simulink model "NewTapWithdrawalCircuit"  (R2016b)
settings: Solver=VariableStepAuto  StartTime=0.0  StopTime=30  RelTol=1e-3  EnableMultiTasking=on
(part 1 of 2)
settings Model: Creator=ramin  LastModifiedBy=ramin
settings DataIOCC: LimitDataPoints=on
settings OptimizationCC: LifeSpan=inf
settings DebuggingCC: AllowSymbolicDim=off  SFUnexpectedBacktrackingDiag=warning  SFNoUnconditionalDefaultTransitionDiag=warning  SFExecutionAtInitializationDiag=none
settings ModelReferenceCC: PropagateSignalLabelsOutOfModel=off
settings GRTTargetCC: TargetLangStandard=C89/C90 (ANSI)
settings ConfigComp: CovMetricSettings=dw  CovHtmlReporting=on  CovSaveCumulativeToWorkspaceVar=on  CovSaveSingleToWorkspaceVar=on  CovExternalEMLEnable=off

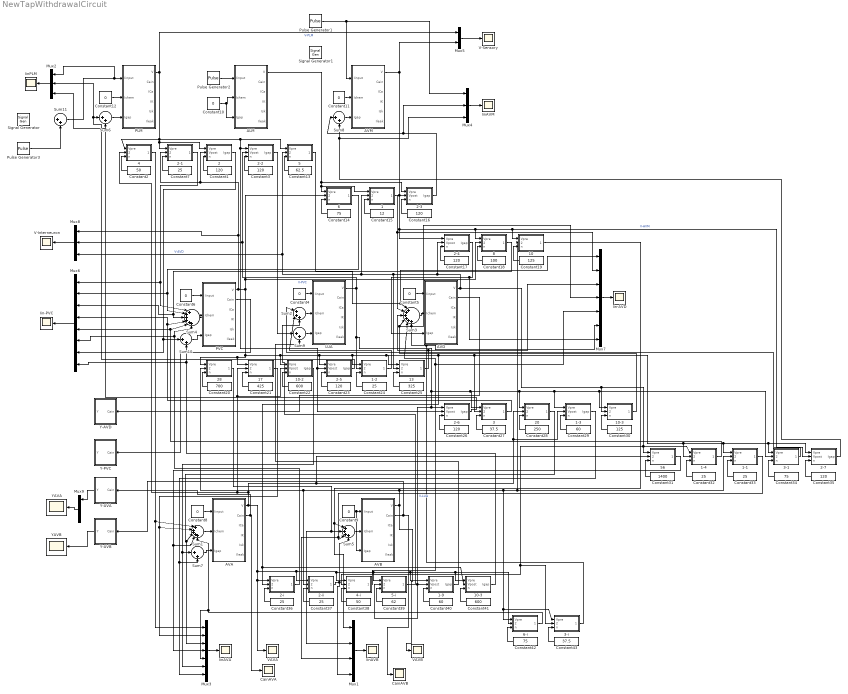
== system NewTapWithdrawalCircuit ==
  1 : Subsystem
  1-1 : Subsystem
  1-2 : Subsystem
  "1-3 " : Subsystem
  1-4 : Subsystem
  1-9 : Subsystem
  10 : Subsystem
  10-2 : Subsystem
  10-3 : Subsystem
  "10-3 " : Subsystem
  13 : Subsystem
  17 : Subsystem
  2 : Subsystem
  2-1 : Subsystem
  2-2 : Subsystem
  2-3 : Subsystem
  2-4 : Subsystem
  2-5 : Subsystem
  2-6 : Subsystem
  2-7 : Subsystem
  2-i : Subsystem
  2-ii : Subsystem
  20 : Subsystem
  28 : Subsystem
  3 : Subsystem
  3-1 : Subsystem
  3-i : Subsystem
  4 : Subsystem
  4-i : Subsystem
  5 : Subsystem
  5-i : Subsystem
  56 : Subsystem
  6 : Subsystem
  6-i : Subsystem
  8 : Subsystem
  ALM : Subsystem
  AVA : Subsystem
  AVB : Subsystem
  AVD : Subsystem
  AVM : Subsystem
  CainAVA : Scope
  CainAVB : Scope
  Constant{1,3,16..17,23,26,35} (7 alike) : Constant  Value=120
  Constant{4..6,8..12} (8 alike) : Constant  Value=0
  Constant13 : Constant  Value=62.5
  Constant14 : Constant  Value=75
  Constant15 : Constant  Value=12
  Constant18 : Constant  Value=100
  Constant19 : Constant  Value=125
  Constant2 : Constant  Value=50
  Constant20 : Constant  Value=700
  Constant21 : Constant  Value=425
  Constant22 : Constant  Value=600
  Constant{7,24,32..33,36..37} (6 alike) : Constant  Value=25
  Constant25 : Constant  Value=325
  Constant27 : Constant  Value=37.5
  Constant28 : Constant  Value=250
  Constant29 : Constant  Value=60
  Constant30 : Constant  Value=125
  Constant31 : Constant  Value=1400
  Constant34 : Constant  Value=75
  Constant38 : Constant  Value=50
  Constant39 : Constant  Value=62
  Constant40 : Constant  Value=60
  Constant41 : Constant  Value=600
  Constant42 : Constant  Value=75
  Constant43 : Constant  Value=37.5
  Iin-AVD : Scope
  Iin-PVC : Scope
  IinAVA : Scope
  IinAVB : Scope
  IinAVM : Scope
  IinPLM : Scope
  LUA : Subsystem
  Mux1 : Mux
  Mux2 : Mux  Inputs=3
  Mux3 : Mux  Inputs=7
  Mux4 : Mux  Inputs=3
  Mux5 : Mux  Inputs=2
  Mux6 : Mux  Inputs=8
  Mux7 : Mux  Inputs=7
  Mux8 : Mux  Inputs=3
  Mux9 : Mux
  PLM : Subsystem
  PVC : Subsystem
  Pulse Generator1 : DiscretePulseGenerator  PulseType=Time based  Amplitude=10000  Period=20  PulseWidth=30  PhaseDelay=2
  Pulse Generator2 : DiscretePulseGenerator  PulseType=Time based  Amplitude=0  Period=12  PulseWidth=30  PhaseDelay=2
  Pulse Generator3 : DiscretePulseGenerator  PulseType=Time based  Amplitude=0  Period=12  PulseWidth=30  PhaseDelay=2
  Signal Generator : SignalGenerator  WaveForm=random  Amplitude=50000  Frequency=500
  Signal Generator1 : SignalGenerator  WaveForm=random  Amplitude=50000  Frequency=500
  Sum1 : Sum  Inputs=|+++++
  Sum{6..11} (6 alike) : Sum  Inputs=|++
  Sum2 : Sum  Inputs=|+++
  Sum3 : Sum  Inputs=|++++++
  Sum4 : Sum  Inputs=|++++++
  Sum5 : Sum  Inputs=|++++
  V-Interneuron : Scope
  V-Sensory : Scope
  VAVA : Scope
  VAVB : Scope
  Y-AVA : Subsystem
  Y-AVB : Subsystem
  Y-AVD : Subsystem
  Y-PVC : Subsystem
  YAVA : Scope
  YAVB : Scope
  wires:
  Constant7/1 -> 2-1/3(n)
  Sum4/1 -> PVC/2(Ichem)
  2-1/1(Ichem) -> Sum4/1, Mux6/1
  Constant1/1 -> 2/3(n)
  2/1(Igap) -> Mux6/7, Sum10/1
  Constant2/1 -> 4/3(n)
  Sum1/1 -> AVA/2(Ichem)
  4/1(Ichem) -> Mux3/1, Sum1/1
  LUA/1(V) -> Mux8/2, 2-2/2(Vpost), 5-i/2(Vpost), 1-9/2(Vpost), 2-6/1(Vpre), 20/1(Vpre), 3-1/2(Vpost), "10-3 "/1(Vpre), "1-3 "/1(Vpre), 3/1(Vpre), 1-2/2(Vpost)  "V-LUA"
  Sum2/1 -> LUA/2(Ichem)
  2-2/1(Igap) -> Sum9/1
  Constant3/1 -> 2-2/3(n)
  Sum11/1 -> Mux2/1, PLM/1(Iinput)
  Sum3/1 -> AVD/2(Ichem)
  5/1(Ichem) -> Mux7/1, Sum3/1
  Constant5/1 -> AVD/1(Iinput)
  Constant4/1 -> LUA/1(Iinput)
  Constant6/1 -> PVC/1(Iinput)
  Constant8/1 -> AVA/1(Iinput)
  Constant9/1 -> AVB/3(Igap), AVB/1(Iinput)
  Pulse Generator2/1 -> ALM/1(Iinput)
  Constant11/1 -> AVM/2(Ichem)
  Constant12/1 -> PLM/2(Ichem)
  Sum5/1 -> AVB/2(Ichem)
  Constant13/1 -> 5/3(n)
  ALM/1(V) -> 2-3/1(Vpre), 1/1(Vpre), 6/1(Vpre)
  6/1(Ichem) -> Sum4/2, Mux6/2
  Constant14/1 -> 6/3(n)
  1/1(Ichem) -> Sum3/2, Mux7/2
  Constant15/1 -> 1/3(n)
  Constant16/1 -> 2-3/3(n)
  AVM/1(V) -> 2-7/2(Vpost), 10/1(Vpre), 8/1(Vpre), 2-4/1(Vpre), 2-3/2(Vpost), Mux5/2  "V-AVM"
  Constant17/1 -> 2-4/3(n)
  2-4/1(Igap) -> Mux7/7, AVD/3(Igap)
  Constant18/1 -> 8/3(n)
  8/1(Ichem) -> Sum4/3, Mux6/3
  Constant19/1 -> 10/3(n)
  10/1(Ichem) -> Mux1/1, Sum5/1
  AVB/1(V) -> 2-ii/2(Vpost), 28/2(Vpost), 3-i/1(Vpre), 6-i/1(Vpre), 1-1/2(Vpost), 10/2(Vpost), VAVB/1
  Constant20/1 -> 28/3(n)
  28/1(Ichem) -> Sum5/2, Mux1/2
  Constant21/1 -> 17/3(n)
  17/1(Ichem) -> Mux3/2, Sum1/2
  Constant22/1 -> 10-2/3(n)
  10-2/1(Igap) -> Mux3/6, Sum7/1
  PLM/1(V) -> 2-2/1(Vpre), 2-6/2(Vpost), 2-5/2(Vpost), 5/1(Vpre), 4/1(Vpre), 2-1/1(Vpre), 2/1(Vpre), Mux5/1  "V-PLM"
  Constant23/1 -> 2-5/3(n)
  2-5/1(Igap) -> Mux2/2, Sum6/1
  Constant24/1 -> 1-2/3(n)
  1-2/1(Ichem) -> Sum2/2
  Constant25/1 -> 13/3(n)
  Constant26/1 -> 2-6/3(n)
  2-6/1(Igap) -> Mux2/3, Sum6/2
  Constant27/1 -> 3/3(n)
  3/1(Ichem) -> Mux6/4, Sum4/4
  Constant28/1 -> 20/3(n)
  20/1(Ichem) -> Sum1/3, Mux3/3
  Constant29/1 -> "1-3 "/3(n)
  "1-3 "/1(Igap) -> Mux3/7, Sum7/2
  Sum7/1 -> AVA/3(Igap)
  Constant30/1 -> "10-3 "/3(n)
  "10-3 "/1(Ichem) -> Mux7/4, Sum3/4
  AVA/1(V) -> 56/2(Vpost), "1-3 "/2(Vpost), 20/2(Vpost), 10-2/2(Vpost), 17/2(Vpost), 4/2(Vpost), 2-ii/1(Vpre), 4-i/1(Vpre), 5-i/1(Vpre), 1-9/1(Vpre), 6-i/2(Vpost), 10-3/1(Vpre), 2-i/1(Vpre), VAVA/1
  Constant31/1 -> 56/3(n)
  56/1(Ichem) -> Mux3/4, Sum1/4
  1-4/1(Ichem) -> Mux6/5, Sum4/5
  Constant32/1 -> 1-4/3(n)
  Constant33/1 -> 1-1/3(n)
  1-1/1(Ichem) -> Mux1/3, Sum5/3
  Constant34/1 -> 3-1/3(n)
  3-1/1(Ichem) -> Sum2/1
  Sum6/1 -> PLM/3(Igap)
  Sum8/1 -> AVM/3(Igap)
  Constant35/1 -> 2-7/3(n)
  2-7/1(Igap) -> Mux4/3, Sum8/2
  Constant36/1 -> 2-i/3(n)
  2-i/1(Ichem) -> Mux6/6, Sum4/6
  Constant37/1 -> 2-ii/3(n)
  2-ii/1(Ichem) -> Mux1/4, Sum5/4
  Constant38/1 -> 4-i/3(n)
  4-i/1(Ichem) -> Mux7/5, Sum3/5
  5-i/1(Ichem) -> Sum2/3
  Constant39/1 -> 5-i/3(n)
  Sum9/1 -> LUA/3(Igap)
  1-9/1(Igap) -> Sum9/2
  Constant40/1 -> 1-9/3(n)
  Constant41/1 -> 10-3/3(n)
  Sum10/1 -> PVC/3(Igap)
  10-3/1(Igap) -> Sum10/2, Mux6/8
  Constant42/1 -> 6-i/3(n)
  6-i/1(Ichem) -> Mux3/5, Sum1/5
  3-i/1(Ichem) -> Sum3/6, Mux7/6
  Constant43/1 -> 3-i/3(n)
  Mux3/1 -> IinAVA/1
  Mux1/1 -> IinAVB/1
  AVA/2("Cain ") -> Y-AVA/1(Cain), CainAVA/1
  AVB/2("Cain ") -> Y-AVB/1(Cain), CainAVB/1
  Constant10/1 -> ALM/3(Igap), ALM/2(Ichem)
  Mux2/1 -> IinPLM/1
  Mux4/1 -> IinAVM/1
  2-3/1(Igap) -> Mux4/2, Sum8/1
  Mux5/1 -> V-Sensory/1
  Mux6/1 -> Iin-PVC/1
  Mux7/1 -> Iin-AVD/1
  13/1(Ichem) -> Mux7/3, Sum3/3
  Mux8/1 -> V-Interneuron/1
  PVC/1(V) -> Mux8/1, 2-1/2(Vpost), 2/2(Vpost), 8/2(Vpost), 6/2(Vpost), 17/1(Vpre), 28/1(Vpre), 2-5/1(Vpre), 2-i/2(Vpost), 10-3/2(Vpost), 3/2(Vpost), 2-7/1(Vpre), 3-1/1(Vpre), 1-1/1(Vpre), 1-4/2(Vpost), 13/1(Vpre), 1-2/1(Vpre), 10-2/1(Vpre)  "V-PVC"
  AVD/1(V) -> 1-4/1(Vpre), 3-i/2(Vpost), 4-i/2(Vpost), 56/1(Vpre), "10-3 "/2(Vpost), 2-4/2(Vpost), 1/2(Vpost), Mux8/3, 5/2(Vpost), 13/2(Vpost)  "V-AVD"
  Y-AVA/1(Y) -> Mux9/1
  Y-AVB/1(Y) -> YAVB/1
  Mux9/1 -> YAVA/1
  PVC/2("Cain ") -> Y-PVC/1(Cain)
  AVD/2("Cain ") -> Y-AVD/1(Cain)
  Pulse Generator1/1 -> AVM/1(Iinput), Mux4/1
  Pulse Generator3/1 -> Sum11/2

== system NewTapWithdrawalCircuit/1 ==
  Vpre : Inport
  Vpost : Inport  Port=2
  n : Inport  Port=3
  Divide1 : Product  Inputs=*/
  Divide2 : Product  Inputs=*/
  Echem : Constant  Value=-90
  Product2 : Product
  Sum6 : Sum  Inputs=|+-
  Sum7 : Sum  Inputs=|++
  Sum8 : Sum  Inputs=|+-
  Vrange : Constant  Value=3
  Vshift : Constant  Value=-30
  betaK1 : Math  SaturateOnIntegerOverflow=on
  c111 : Constant
  Ichem : Outport
  wires:
  Echem/1 -> Sum6/1
  n/1 -> Product2/2
  Sum6/1 -> Product2/1
  Product2/1 -> Divide1/1
  betaK1/1 -> Sum7/1
  c111/1 -> Sum7/2
  Vshift/1 -> Sum8/1
  Vpre/1 -> Sum8/2  "vpre"
  Sum8/1 -> Divide2/1
  Vrange/1 -> Divide2/2
  Divide2/1 -> betaK1/1
  Sum7/1 -> Divide1/2
  Divide1/1 -> Ichem/1  "Ichem"
  Vpost/1 -> Sum6/2

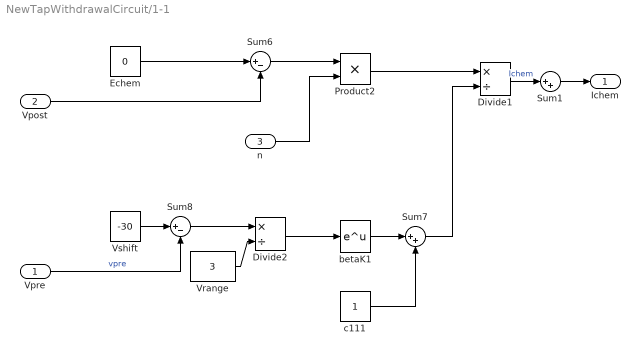
== system NewTapWithdrawalCircuit/1-1 ==
  Vpre : Inport
  Vpost : Inport  Port=2
  n : Inport  Port=3
  Divide1 : Product  Inputs=*/
  Divide2 : Product  Inputs=*/
  Echem : Constant  Value=0
  Product2 : Product
  Sum1 : Sum  Inputs=|++
  Sum6 : Sum  Inputs=|+-
  Sum7 : Sum  Inputs=|++
  Sum8 : Sum  Inputs=|+-
  Vrange : Constant  Value=3
  Vshift : Constant  Value=-30
  betaK1 : Math  SaturateOnIntegerOverflow=on
  c111 : Constant
  Ichem : Outport
  wires:
  Echem/1 -> Sum6/1
  n/1 -> Product2/2
  Sum6/1 -> Product2/1
  Product2/1 -> Divide1/1
  betaK1/1 -> Sum7/1
  c111/1 -> Sum7/2
  Vshift/1 -> Sum8/1
  Vpre/1 -> Sum8/2  "vpre"
  Sum8/1 -> Divide2/1
  Vrange/1 -> Divide2/2
  Divide2/1 -> betaK1/1
  Sum7/1 -> Divide1/2
  Divide1/1 -> Sum1/1  "Ichem"
  Vpost/1 -> Sum6/2
  Sum1/1 -> Ichem/1

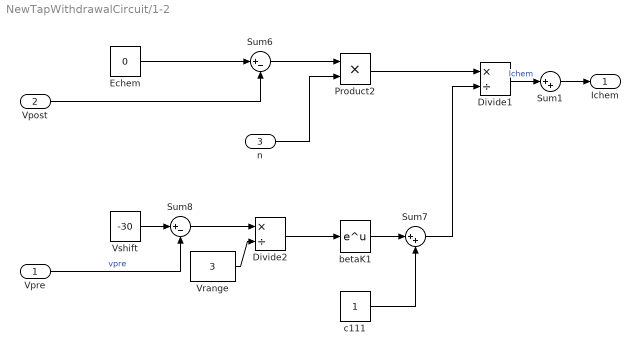
== system NewTapWithdrawalCircuit/1-2 ==
  Vpre : Inport
  Vpost : Inport  Port=2
  n : Inport  Port=3
  Divide1 : Product  Inputs=*/
  Divide2 : Product  Inputs=*/
  Echem : Constant  Value=0
  Product2 : Product
  Sum1 : Sum  Inputs=|++
  Sum6 : Sum  Inputs=|+-
  Sum7 : Sum  Inputs=|++
  Sum8 : Sum  Inputs=|+-
  Vrange : Constant  Value=3
  Vshift : Constant  Value=-30
  betaK1 : Math  SaturateOnIntegerOverflow=on
  c111 : Constant
  Ichem : Outport
  wires:
  Echem/1 -> Sum6/1
  n/1 -> Product2/2
  Sum6/1 -> Product2/1
  Product2/1 -> Divide1/1
  betaK1/1 -> Sum7/1
  c111/1 -> Sum7/2
  Vshift/1 -> Sum8/1
  Vpre/1 -> Sum8/2  "vpre"
  Sum8/1 -> Divide2/1
  Vrange/1 -> Divide2/2
  Divide2/1 -> betaK1/1
  Sum7/1 -> Divide1/2
  Divide1/1 -> Sum1/1  "Ichem"
  Vpost/1 -> Sum6/2
  Sum1/1 -> Ichem/1

== system NewTapWithdrawalCircuit/1-3  ==
  Vpre : Inport
  Vpost : Inport  Port=2
  n : Inport  Port=3
  Ggap : Constant  Value=1.02
  Product2 : Product  Inputs=3
  Sum6 : Sum  Inputs=|+-
  Igap : Outport
  wires:
  Vpre/1 -> Sum6/1
  n/1 -> Product2/2
  Sum6/1 -> Product2/1
  Product2/1 -> Igap/1  "Igap"
  Vpost/1 -> Sum6/2
  Ggap/1 -> Product2/3

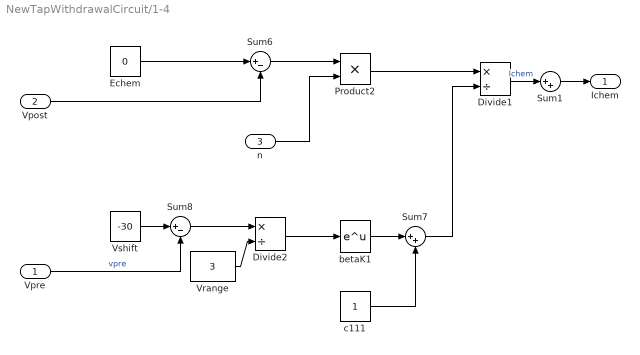
== system NewTapWithdrawalCircuit/1-4 ==
  Vpre : Inport
  Vpost : Inport  Port=2
  n : Inport  Port=3
  Divide1 : Product  Inputs=*/
  Divide2 : Product  Inputs=*/
  Echem : Constant  Value=0
  Product2 : Product
  Sum1 : Sum  Inputs=|++
  Sum6 : Sum  Inputs=|+-
  Sum7 : Sum  Inputs=|++
  Sum8 : Sum  Inputs=|+-
  Vrange : Constant  Value=3
  Vshift : Constant  Value=-30
  betaK1 : Math  SaturateOnIntegerOverflow=on
  c111 : Constant
  Ichem : Outport
  wires:
  Echem/1 -> Sum6/1
  n/1 -> Product2/2
  Sum6/1 -> Product2/1
  Product2/1 -> Divide1/1
  betaK1/1 -> Sum7/1
  c111/1 -> Sum7/2
  Vshift/1 -> Sum8/1
  Vpre/1 -> Sum8/2  "vpre"
  Sum8/1 -> Divide2/1
  Vrange/1 -> Divide2/2
  Divide2/1 -> betaK1/1
  Sum7/1 -> Divide1/2
  Divide1/1 -> Sum1/1  "Ichem"
  Vpost/1 -> Sum6/2
  Sum1/1 -> Ichem/1

== system NewTapWithdrawalCircuit/1-9 ==
  Vpre : Inport
  Vpost : Inport  Port=2
  n : Inport  Port=3
  Ggap : Constant  Value=1.02
  Product2 : Product  Inputs=3
  Sum6 : Sum  Inputs=|+-
  Igap : Outport
  wires:
  Vpre/1 -> Sum6/1
  n/1 -> Product2/2
  Sum6/1 -> Product2/1
  Product2/1 -> Igap/1  "Igap"
  Vpost/1 -> Sum6/2
  Ggap/1 -> Product2/3

== system NewTapWithdrawalCircuit/10 ==
  Vpre : Inport
  Vpost : Inport  Port=2
  n : Inport  Port=3
  Divide1 : Product  Inputs=*/
  Divide2 : Product  Inputs=*/
  Echem : Constant  Value=-90
  Product2 : Product
  Sum6 : Sum  Inputs=|+-
  Sum7 : Sum  Inputs=|++
  Sum8 : Sum  Inputs=|+-
  Vrange : Constant  Value=3
  Vshift : Constant  Value=-30
  betaK1 : Math  SaturateOnIntegerOverflow=on
  c111 : Constant
  Ichem : Outport
  wires:
  Echem/1 -> Sum6/1
  n/1 -> Product2/2
  Sum6/1 -> Product2/1
  Product2/1 -> Divide1/1
  betaK1/1 -> Sum7/1
  c111/1 -> Sum7/2
  Vshift/1 -> Sum8/1
  Vpre/1 -> Sum8/2  "vpre"
  Sum8/1 -> Divide2/1
  Vrange/1 -> Divide2/2
  Divide2/1 -> betaK1/1
  Sum7/1 -> Divide1/2
  Divide1/1 -> Ichem/1  "Ichem"
  Vpost/1 -> Sum6/2

== system NewTapWithdrawalCircuit/10-2 ==
  Vpre : Inport
  Vpost : Inport  Port=2
  n : Inport  Port=3
  Ggap : Constant  Value=1.02
  Product2 : Product  Inputs=3
  Sum6 : Sum  Inputs=|+-
  Igap : Outport
  wires:
  Vpre/1 -> Sum6/1
  n/1 -> Product2/2
  Sum6/1 -> Product2/1
  Product2/1 -> Igap/1  "Igap"
  Vpost/1 -> Sum6/2
  Ggap/1 -> Product2/3

== system NewTapWithdrawalCircuit/10-3 ==
  Vpre : Inport
  Vpost : Inport  Port=2
  n : Inport  Port=3
  Ggap : Constant  Value=1.02
  Product2 : Product  Inputs=3
  Sum6 : Sum  Inputs=|+-
  Igap : Outport
  wires:
  Vpre/1 -> Sum6/1
  n/1 -> Product2/2
  Sum6/1 -> Product2/1
  Product2/1 -> Igap/1  "Igap"
  Vpost/1 -> Sum6/2
  Ggap/1 -> Product2/3

== system NewTapWithdrawalCircuit/10-3  ==
  Vpre : Inport
  Vpost : Inport  Port=2
  n : Inport  Port=3
  Divide1 : Product  Inputs=*/
  Divide2 : Product  Inputs=*/
  Echem : Constant  Value=-90
  Product2 : Product
  Sum6 : Sum  Inputs=|+-
  Sum7 : Sum  Inputs=|++
  Sum8 : Sum  Inputs=|+-
  Vrange : Constant  Value=3
  Vshift : Constant  Value=-30
  betaK1 : Math  SaturateOnIntegerOverflow=on
  c111 : Constant
  Ichem : Outport
  wires:
  Echem/1 -> Sum6/1
  n/1 -> Product2/2
  Sum6/1 -> Product2/1
  Product2/1 -> Divide1/1
  betaK1/1 -> Sum7/1
  c111/1 -> Sum7/2
  Vshift/1 -> Sum8/1
  Vpre/1 -> Sum8/2  "vpre"
  Sum8/1 -> Divide2/1
  Vrange/1 -> Divide2/2
  Divide2/1 -> betaK1/1
  Sum7/1 -> Divide1/2
  Divide1/1 -> Ichem/1  "Ichem"
  Vpost/1 -> Sum6/2

== system NewTapWithdrawalCircuit/13 ==
  Vpre : Inport
  Vpost : Inport  Port=2
  n : Inport  Port=3
  Divide1 : Product  Inputs=*/
  Divide2 : Product  Inputs=*/
  Echem : Constant  Value=0
  Product2 : Product
  Sum1 : Sum  Inputs=|++
  Sum6 : Sum  Inputs=|+-
  Sum7 : Sum  Inputs=|++
  Sum8 : Sum  Inputs=|+-
  Vrange : Constant  Value=3
  Vshift : Constant  Value=-30
  betaK1 : Math  SaturateOnIntegerOverflow=on
  c111 : Constant
  Ichem : Outport
  wires:
  Echem/1 -> Sum6/1
  n/1 -> Product2/2
  Sum6/1 -> Product2/1
  Product2/1 -> Divide1/1
  betaK1/1 -> Sum7/1
  c111/1 -> Sum7/2
  Vshift/1 -> Sum8/1
  Vpre/1 -> Sum8/2  "vpre"
  Sum8/1 -> Divide2/1
  Vrange/1 -> Divide2/2
  Divide2/1 -> betaK1/1
  Sum7/1 -> Divide1/2
  Divide1/1 -> Sum1/1  "Ichem"
  Vpost/1 -> Sum6/2
  Sum1/1 -> Ichem/1

== system NewTapWithdrawalCircuit/17 ==
  Vpre : Inport
  Vpost : Inport  Port=2
  n : Inport  Port=3
  Divide1 : Product  Inputs=*/
  Divide2 : Product  Inputs=*/
  Echem : Constant  Value=0
  Product2 : Product
  Sum1 : Sum  Inputs=|++
  Sum6 : Sum  Inputs=|+-
  Sum7 : Sum  Inputs=|++
  Sum8 : Sum  Inputs=|+-
  Vrange : Constant  Value=3
  Vshift : Constant  Value=-30
  betaK1 : Math  SaturateOnIntegerOverflow=on
  c111 : Constant
  Ichem : Outport
  wires:
  Echem/1 -> Sum6/1
  n/1 -> Product2/2
  Sum6/1 -> Product2/1
  Product2/1 -> Divide1/1
  betaK1/1 -> Sum7/1
  c111/1 -> Sum7/2
  Vshift/1 -> Sum8/1
  Vpre/1 -> Sum8/2  "vpre"
  Sum8/1 -> Divide2/1
  Vrange/1 -> Divide2/2
  Divide2/1 -> betaK1/1
  Sum7/1 -> Divide1/2
  Divide1/1 -> Sum1/1  "Ichem"
  Vpost/1 -> Sum6/2
  Sum1/1 -> Ichem/1

== system NewTapWithdrawalCircuit/2 ==
  Vpre : Inport
  Vpost : Inport  Port=2
  n : Inport  Port=3
  Ggap : Constant  Value=1.02
  Product2 : Product  Inputs=3
  Sum6 : Sum  Inputs=|+-
  Igap : Outport
  wires:
  Vpre/1 -> Sum6/1
  n/1 -> Product2/2
  Sum6/1 -> Product2/1
  Product2/1 -> Igap/1  "Igap"
  Vpost/1 -> Sum6/2
  Ggap/1 -> Product2/3

== system NewTapWithdrawalCircuit/2-1 ==
  Vpre : Inport
  Vpost : Inport  Port=2
  n : Inport  Port=3
  Divide1 : Product  Inputs=*/
  Divide2 : Product  Inputs=*/
  Echem : Constant  Value=-90
  Product2 : Product
  Sum6 : Sum  Inputs=|+-
  Sum7 : Sum  Inputs=|++
  Sum8 : Sum  Inputs=|+-
  Vrange : Constant  Value=3
  Vshift : Constant  Value=-30
  betaK1 : Math  SaturateOnIntegerOverflow=on
  c111 : Constant
  Ichem : Outport
  wires:
  Echem/1 -> Sum6/1
  n/1 -> Product2/2
  Sum6/1 -> Product2/1
  Product2/1 -> Divide1/1
  betaK1/1 -> Sum7/1
  c111/1 -> Sum7/2
  Vshift/1 -> Sum8/1
  Vpre/1 -> Sum8/2  "vpre"
  Sum8/1 -> Divide2/1
  Vrange/1 -> Divide2/2
  Divide2/1 -> betaK1/1
  Sum7/1 -> Divide1/2
  Divide1/1 -> Ichem/1  "Ichem"
  Vpost/1 -> Sum6/2

== system NewTapWithdrawalCircuit/2-2 ==
  Vpre : Inport
  Vpost : Inport  Port=2
  n : Inport  Port=3
  Ggap : Constant  Value=1.02
  Product2 : Product  Inputs=3
  Sum6 : Sum  Inputs=|+-
  Igap : Outport
  wires:
  Vpre/1 -> Sum6/1
  n/1 -> Product2/2
  Sum6/1 -> Product2/1
  Product2/1 -> Igap/1  "Igap"
  Vpost/1 -> Sum6/2
  Ggap/1 -> Product2/3

== system NewTapWithdrawalCircuit/2-3 ==
  Vpre : Inport
  Vpost : Inport  Port=2
  n : Inport  Port=3
  Ggap : Constant  Value=1.02
  Product2 : Product  Inputs=3
  Sum6 : Sum  Inputs=|+-
  Igap : Outport
  wires:
  Vpre/1 -> Sum6/1
  n/1 -> Product2/2
  Sum6/1 -> Product2/1
  Product2/1 -> Igap/1  "Igap"
  Vpost/1 -> Sum6/2
  Ggap/1 -> Product2/3

== system NewTapWithdrawalCircuit/2-4 ==
  Vpre : Inport
  Vpost : Inport  Port=2
  n : Inport  Port=3
  Ggap : Constant  Value=1.02
  Product2 : Product  Inputs=3
  Sum6 : Sum  Inputs=|+-
  Igap : Outport
  wires:
  Vpre/1 -> Sum6/1
  n/1 -> Product2/2
  Sum6/1 -> Product2/1
  Product2/1 -> Igap/1  "Igap"
  Vpost/1 -> Sum6/2
  Ggap/1 -> Product2/3

== system NewTapWithdrawalCircuit/2-5 ==
  Vpre : Inport
  Vpost : Inport  Port=2
  n : Inport  Port=3
  Ggap : Constant  Value=1.02
  Product2 : Product  Inputs=3
  Sum6 : Sum  Inputs=|+-
  Igap : Outport
  wires:
  Vpre/1 -> Sum6/1
  n/1 -> Product2/2
  Sum6/1 -> Product2/1
  Product2/1 -> Igap/1  "Igap"
  Vpost/1 -> Sum6/2
  Ggap/1 -> Product2/3

== system NewTapWithdrawalCircuit/2-6 ==
  Vpre : Inport
  Vpost : Inport  Port=2
  n : Inport  Port=3
  Ggap : Constant  Value=1.02
  Product2 : Product  Inputs=3
  Sum6 : Sum  Inputs=|+-
  Igap : Outport
  wires:
  Vpre/1 -> Sum6/1
  n/1 -> Product2/2
  Sum6/1 -> Product2/1
  Product2/1 -> Igap/1  "Igap"
  Vpost/1 -> Sum6/2
  Ggap/1 -> Product2/3

== system NewTapWithdrawalCircuit/2-7 ==
  Vpre : Inport
  Vpost : Inport  Port=2
  n : Inport  Port=3
  Ggap : Constant  Value=1.02
  Product2 : Product  Inputs=3
  Sum6 : Sum  Inputs=|+-
  Igap : Outport
  wires:
  Vpre/1 -> Sum6/1
  n/1 -> Product2/2
  Sum6/1 -> Product2/1
  Product2/1 -> Igap/1  "Igap"
  Vpost/1 -> Sum6/2
  Ggap/1 -> Product2/3

== system NewTapWithdrawalCircuit/2-i ==
  Vpre : Inport
  Vpost : Inport  Port=2
  n : Inport  Port=3
  Divide1 : Product  Inputs=*/
  Divide2 : Product  Inputs=*/
  Echem : Constant  Value=-90
  Product2 : Product
  Sum6 : Sum  Inputs=|+-
  Sum7 : Sum  Inputs=|++
  Sum8 : Sum  Inputs=|+-
  Vrange : Constant  Value=3
  Vshift : Constant  Value=-30
  betaK1 : Math  SaturateOnIntegerOverflow=on
  c111 : Constant
  Ichem : Outport
  wires:
  Echem/1 -> Sum6/1
  n/1 -> Product2/2
  Sum6/1 -> Product2/1
  Product2/1 -> Divide1/1
  betaK1/1 -> Sum7/1
  c111/1 -> Sum7/2
  Vshift/1 -> Sum8/1
  Vpre/1 -> Sum8/2  "vpre"
  Sum8/1 -> Divide2/1
  Vrange/1 -> Divide2/2
  Divide2/1 -> betaK1/1
  Sum7/1 -> Divide1/2
  Divide1/1 -> Ichem/1  "Ichem"
  Vpost/1 -> Sum6/2

== system NewTapWithdrawalCircuit/2-ii ==
  Vpre : Inport
  Vpost : Inport  Port=2
  n : Inport  Port=3
  Divide1 : Product  Inputs=*/
  Divide2 : Product  Inputs=*/
  Echem : Constant  Value=-90
  Product2 : Product
  Sum6 : Sum  Inputs=|+-
  Sum7 : Sum  Inputs=|++
  Sum8 : Sum  Inputs=|+-
  Vrange : Constant  Value=3
  Vshift : Constant  Value=-30
  betaK1 : Math  SaturateOnIntegerOverflow=on
  c111 : Constant
  Ichem : Outport
  wires:
  Echem/1 -> Sum6/1
  n/1 -> Product2/2
  Sum6/1 -> Product2/1
  Product2/1 -> Divide1/1
  betaK1/1 -> Sum7/1
  c111/1 -> Sum7/2
  Vshift/1 -> Sum8/1
  Vpre/1 -> Sum8/2  "vpre"
  Sum8/1 -> Divide2/1
  Vrange/1 -> Divide2/2
  Divide2/1 -> betaK1/1
  Sum7/1 -> Divide1/2
  Divide1/1 -> Ichem/1  "Ichem"
  Vpost/1 -> Sum6/2

== system NewTapWithdrawalCircuit/20 ==
  Vpre : Inport
  Vpost : Inport  Port=2
  n : Inport  Port=3
  Divide1 : Product  Inputs=*/
  Divide2 : Product  Inputs=*/
  Echem : Constant  Value=-90
  Product2 : Product
  Sum6 : Sum  Inputs=|+-
  Sum7 : Sum  Inputs=|++
  Sum8 : Sum  Inputs=|+-
  Vrange : Constant  Value=3
  Vshift : Constant  Value=-30
  betaK1 : Math  SaturateOnIntegerOverflow=on
  c111 : Constant
  Ichem : Outport
  wires:
  Echem/1 -> Sum6/1
  n/1 -> Product2/2
  Sum6/1 -> Product2/1
  Product2/1 -> Divide1/1
  betaK1/1 -> Sum7/1
  c111/1 -> Sum7/2
  Vshift/1 -> Sum8/1
  Vpre/1 -> Sum8/2  "vpre"
  Sum8/1 -> Divide2/1
  Vrange/1 -> Divide2/2
  Divide2/1 -> betaK1/1
  Sum7/1 -> Divide1/2
  Divide1/1 -> Ichem/1  "Ichem"
  Vpost/1 -> Sum6/2

== system NewTapWithdrawalCircuit/28 ==
  Vpre : Inport
  Vpost : Inport  Port=2
  n : Inport  Port=3
  Divide1 : Product  Inputs=*/
  Divide2 : Product  Inputs=*/
  Echem : Constant  Value=0
  Product2 : Product
  Sum1 : Sum  Inputs=|++
  Sum6 : Sum  Inputs=|+-
  Sum7 : Sum  Inputs=|++
  Sum8 : Sum  Inputs=|+-
  Vrange : Constant  Value=3
  Vshift : Constant  Value=-30
  betaK1 : Math  SaturateOnIntegerOverflow=on
  c111 : Constant
  Ichem : Outport
  wires:
  Echem/1 -> Sum6/1
  n/1 -> Product2/2
  Sum6/1 -> Product2/1
  Product2/1 -> Divide1/1
  betaK1/1 -> Sum7/1
  c111/1 -> Sum7/2
  Vshift/1 -> Sum8/1
  Vpre/1 -> Sum8/2  "vpre"
  Sum8/1 -> Divide2/1
  Vrange/1 -> Divide2/2
  Divide2/1 -> betaK1/1
  Sum7/1 -> Divide1/2
  Divide1/1 -> Sum1/1  "Ichem"
  Vpost/1 -> Sum6/2
  Sum1/1 -> Ichem/1

== system NewTapWithdrawalCircuit/3 ==
  Vpre : Inport
  Vpost : Inport  Port=2
  n : Inport  Port=3
  Divide1 : Product  Inputs=*/
  Divide2 : Product  Inputs=*/
  Echem : Constant  Value=-90
  Product2 : Product
  Sum6 : Sum  Inputs=|+-
  Sum7 : Sum  Inputs=|++
  Sum8 : Sum  Inputs=|+-
  Vrange : Constant  Value=3
  Vshift : Constant  Value=-30
  betaK1 : Math  SaturateOnIntegerOverflow=on
  c111 : Constant
  Ichem : Outport
  wires:
  Echem/1 -> Sum6/1
  n/1 -> Product2/2
  Sum6/1 -> Product2/1
  Product2/1 -> Divide1/1
  betaK1/1 -> Sum7/1
  c111/1 -> Sum7/2
  Vshift/1 -> Sum8/1
  Vpre/1 -> Sum8/2  "vpre"
  Sum8/1 -> Divide2/1
  Vrange/1 -> Divide2/2
  Divide2/1 -> betaK1/1
  Sum7/1 -> Divide1/2
  Divide1/1 -> Ichem/1  "Ichem"
  Vpost/1 -> Sum6/2

== system NewTapWithdrawalCircuit/3-1 ==
  Vpre : Inport
  Vpost : Inport  Port=2
  n : Inport  Port=3
  Divide1 : Product  Inputs=*/
  Divide2 : Product  Inputs=*/
  Echem : Constant  Value=0
  Product2 : Product
  Sum1 : Sum  Inputs=|++
  Sum6 : Sum  Inputs=|+-
  Sum7 : Sum  Inputs=|++
  Sum8 : Sum  Inputs=|+-
  Vrange : Constant  Value=3
  Vshift : Constant  Value=-30
  betaK1 : Math  SaturateOnIntegerOverflow=on
  c111 : Constant
  Ichem : Outport
  wires:
  Echem/1 -> Sum6/1
  n/1 -> Product2/2
  Sum6/1 -> Product2/1
  Product2/1 -> Divide1/1
  betaK1/1 -> Sum7/1
  c111/1 -> Sum7/2
  Vshift/1 -> Sum8/1
  Vpre/1 -> Sum8/2  "vpre"
  Sum8/1 -> Divide2/1
  Vrange/1 -> Divide2/2
  Divide2/1 -> betaK1/1
  Sum7/1 -> Divide1/2
  Divide1/1 -> Sum1/1  "Ichem"
  Vpost/1 -> Sum6/2
  Sum1/1 -> Ichem/1

== system NewTapWithdrawalCircuit/3-i ==
  Vpre : Inport
  Vpost : Inport  Port=2
  n : Inport  Port=3
  Divide1 : Product  Inputs=*/
  Divide2 : Product  Inputs=*/
  Echem : Constant  Value=-90
  Product2 : Product
  Sum6 : Sum  Inputs=|+-
  Sum7 : Sum  Inputs=|++
  Sum8 : Sum  Inputs=|+-
  Vrange : Constant  Value=3
  Vshift : Constant  Value=-30
  betaK1 : Math  SaturateOnIntegerOverflow=on
  c111 : Constant
  Ichem : Outport
  wires:
  Echem/1 -> Sum6/1
  n/1 -> Product2/2
  Sum6/1 -> Product2/1
  Product2/1 -> Divide1/1
  betaK1/1 -> Sum7/1
  c111/1 -> Sum7/2
  Vshift/1 -> Sum8/1
  Vpre/1 -> Sum8/2  "vpre"
  Sum8/1 -> Divide2/1
  Vrange/1 -> Divide2/2
  Divide2/1 -> betaK1/1
  Sum7/1 -> Divide1/2
  Divide1/1 -> Ichem/1  "Ichem"
  Vpost/1 -> Sum6/2

== system NewTapWithdrawalCircuit/4 ==
  Vpre : Inport
  Vpost : Inport  Port=2
  n : Inport  Port=3
  Divide1 : Product  Inputs=*/
  Divide2 : Product  Inputs=*/
  Echem : Constant  Value=-90
  Product2 : Product
  Sum6 : Sum  Inputs=|+-
  Sum7 : Sum  Inputs=|++
  Sum8 : Sum  Inputs=|+-
  Vrange : Constant  Value=3
  Vshift : Constant  Value=-30
  betaK1 : Math  SaturateOnIntegerOverflow=on
  c111 : Constant
  Ichem : Outport
  wires:
  Echem/1 -> Sum6/1
  n/1 -> Product2/2
  Sum6/1 -> Product2/1
  Product2/1 -> Divide1/1
  betaK1/1 -> Sum7/1
  c111/1 -> Sum7/2
  Vshift/1 -> Sum8/1
  Vpre/1 -> Sum8/2  "vpre"
  Sum8/1 -> Divide2/1
  Vrange/1 -> Divide2/2
  Divide2/1 -> betaK1/1
  Sum7/1 -> Divide1/2
  Divide1/1 -> Ichem/1  "Ichem"
  Vpost/1 -> Sum6/2

== system NewTapWithdrawalCircuit/4-i ==
  Vpre : Inport
  Vpost : Inport  Port=2
  n : Inport  Port=3
  Divide1 : Product  Inputs=*/
  Divide2 : Product  Inputs=*/
  Echem : Constant  Value=-90
  Product2 : Product
  Sum6 : Sum  Inputs=|+-
  Sum7 : Sum  Inputs=|++
  Sum8 : Sum  Inputs=|+-
  Vrange : Constant  Value=3
  Vshift : Constant  Value=-30
  betaK1 : Math  SaturateOnIntegerOverflow=on
  c111 : Constant
  Ichem : Outport
  wires:
  Echem/1 -> Sum6/1
  n/1 -> Product2/2
  Sum6/1 -> Product2/1
  Product2/1 -> Divide1/1
  betaK1/1 -> Sum7/1
  c111/1 -> Sum7/2
  Vshift/1 -> Sum8/1
  Vpre/1 -> Sum8/2  "vpre"
  Sum8/1 -> Divide2/1
  Vrange/1 -> Divide2/2
  Divide2/1 -> betaK1/1
  Sum7/1 -> Divide1/2
  Divide1/1 -> Ichem/1  "Ichem"
  Vpost/1 -> Sum6/2

== system NewTapWithdrawalCircuit/5 ==
  Vpre : Inport
  Vpost : Inport  Port=2
  n : Inport  Port=3
  Divide1 : Product  Inputs=*/
  Divide2 : Product  Inputs=*/
  Echem : Constant  Value=-90
  Product2 : Product
  Sum6 : Sum  Inputs=|+-
  Sum7 : Sum  Inputs=|++
  Sum8 : Sum  Inputs=|+-
  Vrange : Constant  Value=3
  Vshift : Constant  Value=-30
  betaK1 : Math  SaturateOnIntegerOverflow=on
  c111 : Constant
  Ichem : Outport
  wires:
  Echem/1 -> Sum6/1
  n/1 -> Product2/2
  Sum6/1 -> Product2/1
  Product2/1 -> Divide1/1
  betaK1/1 -> Sum7/1
  c111/1 -> Sum7/2
  Vshift/1 -> Sum8/1
  Vpre/1 -> Sum8/2  "vpre"
  Sum8/1 -> Divide2/1
  Vrange/1 -> Divide2/2
  Divide2/1 -> betaK1/1
  Sum7/1 -> Divide1/2
  Divide1/1 -> Ichem/1  "Ichem"
  Vpost/1 -> Sum6/2

== system NewTapWithdrawalCircuit/5-i ==
  Vpre : Inport
  Vpost : Inport  Port=2
  n : Inport  Port=3
  Divide1 : Product  Inputs=*/
  Divide2 : Product  Inputs=*/
  Echem : Constant  Value=-90
  Product2 : Product
  Sum6 : Sum  Inputs=|+-
  Sum7 : Sum  Inputs=|++
  Sum8 : Sum  Inputs=|+-
  Vrange : Constant  Value=3
  Vshift : Constant  Value=-30
  betaK1 : Math  SaturateOnIntegerOverflow=on
  c111 : Constant
  Ichem : Outport
  wires:
  Echem/1 -> Sum6/1
  n/1 -> Product2/2
  Sum6/1 -> Product2/1
  Product2/1 -> Divide1/1
  betaK1/1 -> Sum7/1
  c111/1 -> Sum7/2
  Vshift/1 -> Sum8/1
  Vpre/1 -> Sum8/2  "vpre"
  Sum8/1 -> Divide2/1
  Vrange/1 -> Divide2/2
  Divide2/1 -> betaK1/1
  Sum7/1 -> Divide1/2
  Divide1/1 -> Ichem/1  "Ichem"
  Vpost/1 -> Sum6/2

== system NewTapWithdrawalCircuit/56 ==
  Vpre : Inport
  Vpost : Inport  Port=2
  n : Inport  Port=3
  Divide1 : Product  Inputs=*/
  Divide2 : Product  Inputs=*/
  Echem : Constant  Value=0
  Product2 : Product
  Sum1 : Sum  Inputs=|++
  Sum6 : Sum  Inputs=|+-
  Sum7 : Sum  Inputs=|++
  Sum8 : Sum  Inputs=|+-
  Vrange : Constant  Value=3
  Vshift : Constant  Value=-30
  betaK1 : Math  SaturateOnIntegerOverflow=on
  c111 : Constant
  Ichem : Outport
  wires:
  Echem/1 -> Sum6/1
  n/1 -> Product2/2
  Sum6/1 -> Product2/1
  Product2/1 -> Divide1/1
  betaK1/1 -> Sum7/1
  c111/1 -> Sum7/2
  Vshift/1 -> Sum8/1
  Vpre/1 -> Sum8/2  "vpre"
  Sum8/1 -> Divide2/1
  Vrange/1 -> Divide2/2
  Divide2/1 -> betaK1/1
  Sum7/1 -> Divide1/2
  Divide1/1 -> Sum1/1  "Ichem"
  Vpost/1 -> Sum6/2
  Sum1/1 -> Ichem/1

== system NewTapWithdrawalCircuit/6 ==
  Vpre : Inport
  Vpost : Inport  Port=2
  n : Inport  Port=3
  Divide1 : Product  Inputs=*/
  Divide2 : Product  Inputs=*/
  Echem : Constant  Value=-90
  Product2 : Product
  Sum6 : Sum  Inputs=|+-
  Sum7 : Sum  Inputs=|++
  Sum8 : Sum  Inputs=|+-
  Vrange : Constant  Value=3
  Vshift : Constant  Value=-30
  betaK1 : Math  SaturateOnIntegerOverflow=on
  c111 : Constant
  Ichem : Outport
  wires:
  Echem/1 -> Sum6/1
  n/1 -> Product2/2
  Sum6/1 -> Product2/1
  Product2/1 -> Divide1/1
  betaK1/1 -> Sum7/1
  c111/1 -> Sum7/2
  Vshift/1 -> Sum8/1
  Vpre/1 -> Sum8/2  "vpre"
  Sum8/1 -> Divide2/1
  Vrange/1 -> Divide2/2
  Divide2/1 -> betaK1/1
  Sum7/1 -> Divide1/2
  Divide1/1 -> Ichem/1  "Ichem"
  Vpost/1 -> Sum6/2

== system NewTapWithdrawalCircuit/6-i ==
  Vpre : Inport
  Vpost : Inport  Port=2
  n : Inport  Port=3
  Divide1 : Product  Inputs=*/
  Divide2 : Product  Inputs=*/
  Echem : Constant  Value=-90
  Product2 : Product
  Sum6 : Sum  Inputs=|+-
  Sum7 : Sum  Inputs=|++
  Sum8 : Sum  Inputs=|+-
  Vrange : Constant  Value=3
  Vshift : Constant  Value=-30
  betaK1 : Math  SaturateOnIntegerOverflow=on
  c111 : Constant
  Ichem : Outport
  wires:
  Echem/1 -> Sum6/1
  n/1 -> Product2/2
  Sum6/1 -> Product2/1
  Product2/1 -> Divide1/1
  betaK1/1 -> Sum7/1
  c111/1 -> Sum7/2
  Vshift/1 -> Sum8/1
  Vpre/1 -> Sum8/2  "vpre"
  Sum8/1 -> Divide2/1
  Vrange/1 -> Divide2/2
  Divide2/1 -> betaK1/1
  Sum7/1 -> Divide1/2
  Divide1/1 -> Ichem/1  "Ichem"
  Vpost/1 -> Sum6/2

== system NewTapWithdrawalCircuit/8 ==
  Vpre : Inport
  Vpost : Inport  Port=2
  n : Inport  Port=3
  Divide1 : Product  Inputs=*/
  Divide2 : Product  Inputs=*/
  Echem : Constant  Value=-90
  Product2 : Product
  Sum6 : Sum  Inputs=|+-
  Sum7 : Sum  Inputs=|++
  Sum8 : Sum  Inputs=|+-
  Vrange : Constant  Value=3
  Vshift : Constant  Value=-30
  betaK1 : Math  SaturateOnIntegerOverflow=on
  c111 : Constant
  Ichem : Outport
  wires:
  Echem/1 -> Sum6/1
  n/1 -> Product2/2
  Sum6/1 -> Product2/1
  Product2/1 -> Divide1/1
  betaK1/1 -> Sum7/1
  c111/1 -> Sum7/2
  Vshift/1 -> Sum8/1
  Vpre/1 -> Sum8/2  "vpre"
  Sum8/1 -> Divide2/1
  Vrange/1 -> Divide2/2
  Divide2/1 -> betaK1/1
  Sum7/1 -> Divide1/2
  Divide1/1 -> Ichem/1  "Ichem"
  Vpost/1 -> Sum6/2

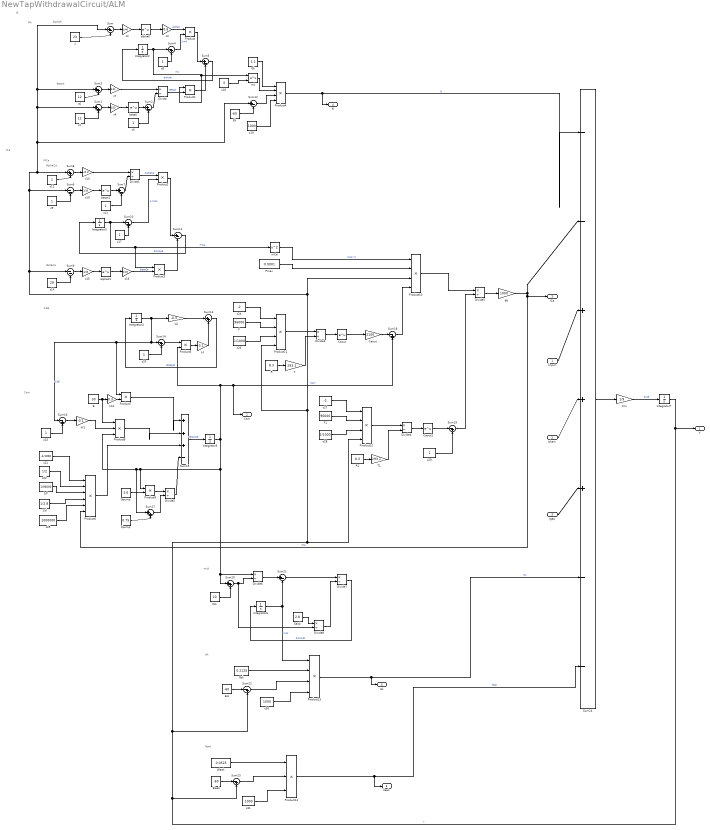
== system NewTapWithdrawalCircuit/ALM ==
  note: Isk
  note: msk
  note: ICa
  note: Cain
  note: CaB
  note: BetaCa
  note: AlphaCa
  note: MCa
  note: IK
  note: Mk
  note: BetaK
  note: AlphaK
  note: Ileak
  Iinput : Inport
  Ichem : Inport  Port=2
  Igap : Inport  Port=3
  1/F : Constant  Value=1/96000
  1/d : Constant  Value=1/2.8
  B : Constant  Value=30
  Caout : Math  SaturateOnIntegerOverflow=on
  "Caout " : Gain  Gain=2100
  Caout1 : Math  SaturateOnIntegerOverflow=on
  "Cm " : Gain  Gain=1/9
  Divide{,1..8} (9 alike) : Product  Inputs=*/
  "Ek " : Constant  Value=-60
  Eleak : Constant  Value=-60
  Esk : Constant  Value=-60
  F : Constant  Value=96000
  F1 : Constant  Value=96000
  "Gk " : Constant  Value=1.1
  Gleak : Constant  Value=0.0525
  Gpump : Constant  Value=3.6
  Gsk : Constant  Value=0.2125
  Integrator2 : Integrator
  Integrator3 : Integrator  InitialCondition=0.001
  Integrator4 : Integrator
  Integrator5 : Integrator
  Integrator6 : Integrator  InitialCondition=1
  Integrator7 : Integrator  InitialCondition=-60
  Kpump : Constant  Value=0.75
  Ksk : Constant  Value=10
  Pmax : Constant  Value=0.0001
  Product{,1..3,5,7,9} (7 alike) : Product
  Product{4,10..13} (5 alike) : Product  Inputs=4
  Product14 : Product  Inputs=3
  Product6 : Product  Inputs=6
  Product8 : Product  Inputs=3
  R : Constant  Value=8.3
  R1 : Constant  Value=8.3
  Saisk : Constant  Value=2.8
  Sum{,2,5,7,11..12,21} (7 alike) : Sum  Inputs=|+-
  Sum{1,3,8,13,17,20} (6 alike) : Sum  Inputs=|++
  Sum{4,10,14,16,18..19,22..23} (8 alike) : Sum  Inputs=|-+
  Sum15 : Sum  Inputs=|+++-
  Sum24 : Sum  Inputs=|--+++--
  Sum6 : Sum  Inputs=|--
  Sum9 : Sum  Inputs=|--
  T : Gain  Gain=293.1
  T1 : Gain  Gain=293.1
  alphaK : Math  SaturateOnIntegerOverflow=on
  alphaK1 : Math  SaturateOnIntegerOverflow=on
  betaK : Math  SaturateOnIntegerOverflow=on
  betaK1 : Math  SaturateOnIntegerOverflow=on
  c : Constant  Value=23
  c1 : Constant  Value=12
  c10 : Gain  Gain=1/10
  c{5,8..9,11..12,17,20,23,29} (9 alike) : Constant
  c13 : Gain  Gain=-0.2
  c14 : Constant  Value=29
  c15 : Gain  Gain=1/10
  c16 : Gain  Gain=0.23
  c18 : Constant  Value=3
  c19 : Constant  Value=1000
  c2 : Gain  Gain=1/46
  c21 : Constant  Value=-1/1000
  c22 : Constant  Value=1/2
  c24 : Constant  Value=-2
  c25 : Constant  Value=1000000
  c26 : Constant  Value=1/1000
  c27 : Constant  Value=-2
  c28 : Constant  Value=1/1000
  c3 : Gain  Gain=0.6
  c30 : Constant  Value=1000
  c31 : Constant  Value=1000
  c4 : Gain  Gain=1/23
  c6 : Constant  Value=12
  c7 : Gain  Gain=0.01
  "gg " : Gain  Gain=1000
  kb : Gain  Gain=-0.3
  kb1 : Gain  Gain=0.3
  kf : Gain  Gain=0.1
  kf1 : Gain  Gain=-0.1
  mCa : Math  Operator=square  SaturateOnIntegerOverflow=on
  mk : Math  Operator=pow  SaturateOnIntegerOverflow=on
  V : Outport
  "Cain " : Outport  Port=2
  ICa : Outport  Port=3
  IK : Outport  Port=4
  Isk : Outport  Port=5
  Ileak : Outport  Port=6
  wires:
  Divide/1 -> Product1/2  "BetaK"
  c10/1 -> betaK1/1
  Sum7/1 -> Divide1/2
  c/1 -> Sum/2
  R/1 -> T/1
  c3/1 -> Product/1  "alphaK"
  c9/1 -> Sum6/2
  c6/1 -> Sum3/2
  Product/1 -> Sum5/1
  Sum1/1 -> c4/1
  c13/1 -> Divide1/1
  Caout1/1 -> Sum19/1
  Eleak/1 -> Sum23/1
  T/1 -> Divide3/2
  Ksk/1 -> Sum20/2
  Product14/1 -> Ileak/1, Sum24/7  "Ileak"
  Sum24/1 -> "Cm "/1
  Esk/1 -> Sum22/1
  "Cm "/1 -> Integrator7/1  "dv/dt"
  Divide3/1 -> Caout/1
  c31/1 -> Product14/3
  Integrator6/1 -> Sum21/2, Product13/1  "msk"
  Sum21/1 -> Divide7/1
  Sum23/1 -> Product14/2
  Divide6/1 -> Sum21/1
  c12/1 -> Sum8/2
  Integrator3/1 -> Product3/1, mCa/1, Sum10/1  "mCa"
  Sum5/1 -> Integrator2/1  "dmk/dt"
  c15/1 -> alphaK1/1
  Sum9/1 -> c15/1
  c2/1 -> alphaK/1
  Sum22/1 -> Product13/3
  Product10/1 -> Divide5/1
  Integrator2/1 -> mk/1, Product1/1, Sum4/1  "mk"
  Divide8/1 -> Divide7/2
  R1/1 -> T1/1
  Caout/1 -> "Caout "/1
  Sum3/1 -> c7/1
  Sum6/1 -> c10/1
  Divide4/1 -> Caout1/1
  c30/1 -> Product13/4
  Gleak/1 -> Product14/1
  c28/1 -> Product12/3
  c11/1 -> Sum7/2
  betaK1/1 -> Sum7/1
  Divide7/1 -> Integrator6/1  "dmsk/dt"
  Ichem/1 -> Sum24/4
  c7/1 -> Divide/1
  Sum14/1 -> Product5/1
  Sum13/1 -> Integrator4/1  "dCaB/dt"
  Integrator5/1 -> Sum20/1, Divide6/1, Product9/1, Sum17/1, Product8/3, "Cain "/1, Sum18/2, Product5/2  "Cain"
  c21/1 -> Product6/1
  c22/1 -> Product6/2
  1/F/1 -> Product6/3
  1/d/1 -> Product6/4
  c25/1 -> Product6/5
  "gg "/1 -> Sum24/2, ICa/1, Product6/6  "ICa"
  B/1 -> Product8/1, kb1/1
  kb1/1 -> Product7/2
  Product7/1 -> Sum15/1
  Product5/1 -> kf/1
  kf/1 -> Sum13/2
  c23/1 -> Sum16/2
  Sum16/1 -> kf1/1
  kf1/1 -> Product8/2
  Product8/1 -> Sum15/2
  Product6/1 -> Sum15/3
  Gpump/1 -> Product9/2
  Product9/1 -> Divide2/1
  Kpump/1 -> Sum17/2
  Sum17/1 -> Divide2/2
  Divide2/1 -> Sum15/4
  Sum15/1 -> Integrator5/1  "dCain/dt"
  mCa/1 -> Product10/1  "mCa^2"
  Pmax/1 -> Product10/2
  c24/1 -> Product11/1
  F/1 -> Product11/2
  c26/1 -> Product11/3
  Integrator7/1 -> V/1, Sum22/2, Product11/4, Product10/3, Sum6/1, Sum1/1, Sum3/1, Sum/1, Sum12/1, Sum8/1, Sum9/1, Product12/4, Sum23/2  "v"
  c14/1 -> Sum9/2
  Saisk/1 -> Divide8/1
  Sum18/1 -> Product10/4
  Iinput/1 -> Sum24/3
  "Caout "/1 -> Sum18/1
  Sum/1 -> c2/1
  Sum8/1 -> c13/1
  c16/1 -> Product3/2  "BetaCa"
  Product11/1 -> Divide3/1
  T1/1 -> Divide4/2
  betaK/1 -> Sum2/1
  c29/1 -> Sum19/2
  Product1/1 -> Sum5/2
  c4/1 -> betaK/1
  alphaK/1 -> c3/1
  alphaK1/1 -> c16/1
  Divide1/1 -> Product2/1  "AlphaCa"
  Sum2/1 -> Divide/2
  Sum4/1 -> Product/2  "1-mk"
  c5/1 -> Sum2/2
  c8/1 -> Sum4/2
  Igap/1 -> Sum24/5
  Product13/1 -> Isk/1, Sum24/6  "Isk"
  Divide5/1 -> "gg "/1
  Sum20/1 -> Divide8/2, Divide6/2
  Gsk/1 -> Product13/2
  Product12/1 -> Divide4/1
  c27/1 -> Product12/1
  F1/1 -> Product12/2
  c1/1 -> Sum1/2
  Sum11/1 -> Integrator3/1  "dmCa/dt"
  c17/1 -> Sum10/2
  "Ek "/1 -> Sum12/2
  Sum10/1 -> Product2/2  "1-mCa"
  Sum12/1 -> Product4/3
  Product3/1 -> Sum11/2
  Product4/1 -> IK/1, Sum24/1  "IK"
  Integrator4/1 -> Product7/1, Sum16/1, Sum14/1, kb/1  "CaB"
  kb/1 -> Sum13/1
  c20/1 -> Sum14/2
  mk/1 -> Product4/2
  "Gk "/1 -> Product4/1
  c19/1 -> Product4/4
  Product2/1 -> Sum11/1
  c18/1 -> mk/2
  Sum19/1 -> Divide5/2

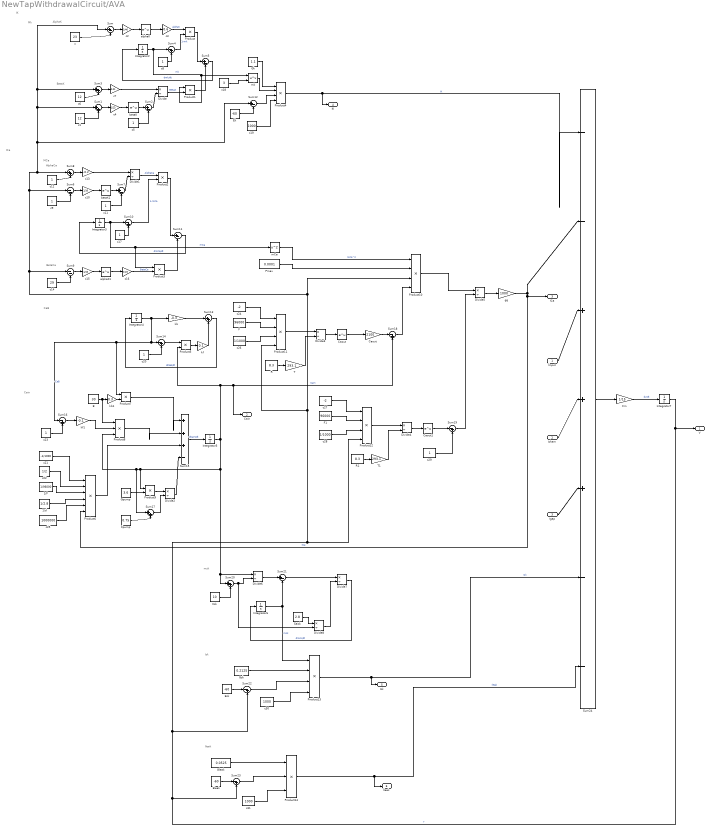
== system NewTapWithdrawalCircuit/AVA ==
  note: Isk
  note: msk
  note: ICa
  note: Cain
  note: CaB
  note: BetaCa
  note: AlphaCa
  note: MCa
  note: IK
  note: Mk
  note: BetaK
  note: AlphaK
  note: Ileak
  Iinput : Inport
  Ichem : Inport  Port=2
  Igap : Inport  Port=3
  1/F : Constant  Value=1/96000
  1/d : Constant  Value=1/2.8
  B : Constant  Value=30
  Caout : Math  SaturateOnIntegerOverflow=on
  "Caout " : Gain  Gain=2100
  Caout1 : Math  SaturateOnIntegerOverflow=on
  "Cm " : Gain  Gain=1/15
  Divide{,1..8} (9 alike) : Product  Inputs=*/
  "Ek " : Constant  Value=-60
  Eleak : Constant  Value=-60
  Esk : Constant  Value=-60
  F : Constant  Value=96000
  F1 : Constant  Value=96000
  "Gk " : Constant  Value=1.1
  Gleak : Constant  Value=0.0525
  Gpump : Constant  Value=3.6
  Gsk : Constant  Value=0.2125
  Integrator2 : Integrator
  Integrator3 : Integrator  InitialCondition=0.001
  Integrator4 : Integrator
  Integrator5 : Integrator
  Integrator6 : Integrator  InitialCondition=1
  Integrator7 : Integrator  InitialCondition=-60
  Kpump : Constant  Value=0.75
  Ksk : Constant  Value=10
  Pmax : Constant  Value=0.0001
  Product{,1..3,5,7,9} (7 alike) : Product
  Product{4,10..13} (5 alike) : Product  Inputs=4
  Product14 : Product  Inputs=3
  Product6 : Product  Inputs=6
  Product8 : Product  Inputs=3
  R : Constant  Value=8.3
  R1 : Constant  Value=8.3
  Saisk : Constant  Value=2.8
  Sum{,2,5,7,11..12,21} (7 alike) : Sum  Inputs=|+-
  Sum{1,3,8,13,17,20} (6 alike) : Sum  Inputs=|++
  Sum{4,10,14,16,18..19,22..23} (8 alike) : Sum  Inputs=|-+
  Sum15 : Sum  Inputs=|+++-
  Sum24 : Sum  Inputs=|--+++--
  Sum6 : Sum  Inputs=|--
  Sum9 : Sum  Inputs=|--
  T : Gain  Gain=293.1
  T1 : Gain  Gain=293.1
  alphaK : Math  SaturateOnIntegerOverflow=on
  alphaK1 : Math  SaturateOnIntegerOverflow=on
  betaK : Math  SaturateOnIntegerOverflow=on
  betaK1 : Math  SaturateOnIntegerOverflow=on
  c : Constant  Value=23
  c1 : Constant  Value=12
  c10 : Gain  Gain=1/10
  c{5,8..9,11..12,17,20,23,29} (9 alike) : Constant
  c13 : Gain  Gain=-0.2
  c14 : Constant  Value=29
  c15 : Gain  Gain=1/10
  c16 : Gain  Gain=0.23
  c18 : Constant  Value=3
  c19 : Constant  Value=1000
  c2 : Gain  Gain=1/46
  c21 : Constant  Value=-1/1000
  c22 : Constant  Value=1/2
  c24 : Constant  Value=-2
  c25 : Constant  Value=1000000
  c26 : Constant  Value=1/1000
  c27 : Constant  Value=-2
  c28 : Constant  Value=1/1000
  c3 : Gain  Gain=0.6
  c30 : Constant  Value=1000
  c31 : Constant  Value=1000
  c4 : Gain  Gain=1/23
  c6 : Constant  Value=12
  c7 : Gain  Gain=0.01
  "gg " : Gain  Gain=1000
  kb : Gain  Gain=-0.3
  kb1 : Gain  Gain=0.3
  kf : Gain  Gain=0.1
  kf1 : Gain  Gain=-0.1
  mCa : Math  Operator=square  SaturateOnIntegerOverflow=on
  mk : Math  Operator=pow  SaturateOnIntegerOverflow=on
  V : Outport
  "Cain " : Outport  Port=2
  ICa : Outport  Port=3
  IK : Outport  Port=4
  Isk : Outport  Port=5
  Ileak : Outport  Port=6
  wires:
  Divide/1 -> Product1/2  "BetaK"
  c10/1 -> betaK1/1
  Sum7/1 -> Divide1/2
  c/1 -> Sum/2
  R/1 -> T/1
  c3/1 -> Product/1  "alphaK"
  c9/1 -> Sum6/2
  c6/1 -> Sum3/2
  Product/1 -> Sum5/1
  Sum1/1 -> c4/1
  c13/1 -> Divide1/1
  Caout1/1 -> Sum19/1
  Eleak/1 -> Sum23/1
  T/1 -> Divide3/2
  Ksk/1 -> Sum20/2
  Product14/1 -> Ileak/1, Sum24/7  "Ileak"
  Sum24/1 -> "Cm "/1
  Esk/1 -> Sum22/1
  "Cm "/1 -> Integrator7/1  "dv/dt"
  Divide3/1 -> Caout/1
  c31/1 -> Product14/3
  Integrator6/1 -> Sum21/2, Product13/1  "msk"
  Sum21/1 -> Divide7/1
  Sum23/1 -> Product14/2
  Divide6/1 -> Sum21/1
  c12/1 -> Sum8/2
  Integrator3/1 -> Product3/1, mCa/1, Sum10/1  "mCa"
  Sum5/1 -> Integrator2/1  "dmk/dt"
  c15/1 -> alphaK1/1
  Sum9/1 -> c15/1
  c2/1 -> alphaK/1
  Sum22/1 -> Product13/3
  Product10/1 -> Divide5/1
  Integrator2/1 -> mk/1, Product1/1, Sum4/1  "mk"
  Divide8/1 -> Divide7/2
  R1/1 -> T1/1
  Caout/1 -> "Caout "/1
  Sum3/1 -> c7/1
  Sum6/1 -> c10/1
  Divide4/1 -> Caout1/1
  c30/1 -> Product13/4
  Gleak/1 -> Product14/1
  c28/1 -> Product12/3
  c11/1 -> Sum7/2
  betaK1/1 -> Sum7/1
  Divide7/1 -> Integrator6/1  "dmsk/dt"
  Ichem/1 -> Sum24/4
  c7/1 -> Divide/1
  Sum14/1 -> Product5/1
  Sum13/1 -> Integrator4/1  "dCaB/dt"
  Integrator5/1 -> Sum20/1, Divide6/1, Product9/1, Sum17/1, Product8/3, "Cain "/1, Sum18/2, Product5/2  "Cain"
  c21/1 -> Product6/1
  c22/1 -> Product6/2
  1/F/1 -> Product6/3
  1/d/1 -> Product6/4
  c25/1 -> Product6/5
  "gg "/1 -> Sum24/2, ICa/1, Product6/6  "ICa"
  B/1 -> Product8/1, kb1/1
  kb1/1 -> Product7/2
  Product7/1 -> Sum15/1
  Product5/1 -> kf/1
  kf/1 -> Sum13/2
  c23/1 -> Sum16/2
  Sum16/1 -> kf1/1
  kf1/1 -> Product8/2
  Product8/1 -> Sum15/2
  Product6/1 -> Sum15/3
  Gpump/1 -> Product9/2
  Product9/1 -> Divide2/1
  Kpump/1 -> Sum17/2
  Sum17/1 -> Divide2/2
  Divide2/1 -> Sum15/4
  Sum15/1 -> Integrator5/1  "dCain/dt"
  mCa/1 -> Product10/1  "mCa^2"
  Pmax/1 -> Product10/2
  c24/1 -> Product11/1
  F/1 -> Product11/2
  c26/1 -> Product11/3
  Integrator7/1 -> V/1, Sum22/2, Product11/4, Product10/3, Sum6/1, Sum1/1, Sum3/1, Sum/1, Sum12/1, Sum8/1, Sum9/1, Product12/4, Sum23/2  "v"
  c14/1 -> Sum9/2
  Saisk/1 -> Divide8/1
  Sum18/1 -> Product10/4
  Iinput/1 -> Sum24/3
  "Caout "/1 -> Sum18/1
  Sum/1 -> c2/1
  Sum8/1 -> c13/1
  c16/1 -> Product3/2  "BetaCa"
  Product11/1 -> Divide3/1
  T1/1 -> Divide4/2
  betaK/1 -> Sum2/1
  c29/1 -> Sum19/2
  Product1/1 -> Sum5/2
  c4/1 -> betaK/1
  alphaK/1 -> c3/1
  alphaK1/1 -> c16/1
  Divide1/1 -> Product2/1  "AlphaCa"
  Sum2/1 -> Divide/2
  Sum4/1 -> Product/2  "1-mk"
  c5/1 -> Sum2/2
  c8/1 -> Sum4/2
  Igap/1 -> Sum24/5
  Product13/1 -> Isk/1, Sum24/6  "Isk"
  Divide5/1 -> "gg "/1
  Sum20/1 -> Divide8/2, Divide6/2
  Gsk/1 -> Product13/2
  Product12/1 -> Divide4/1
  c27/1 -> Product12/1
  F1/1 -> Product12/2
  c1/1 -> Sum1/2
  Sum11/1 -> Integrator3/1  "dmCa/dt"
  c17/1 -> Sum10/2
  "Ek "/1 -> Sum12/2
  Sum10/1 -> Product2/2  "1-mCa"
  Sum12/1 -> Product4/3
  Product3/1 -> Sum11/2
  Product4/1 -> IK/1, Sum24/1  "IK"
  Integrator4/1 -> Product7/1, Sum16/1, Sum14/1, kb/1  "CaB"
  kb/1 -> Sum13/1
  c20/1 -> Sum14/2
  mk/1 -> Product4/2
  "Gk "/1 -> Product4/1
  c19/1 -> Product4/4
  Product2/1 -> Sum11/1
  c18/1 -> mk/2
  Sum19/1 -> Divide5/2

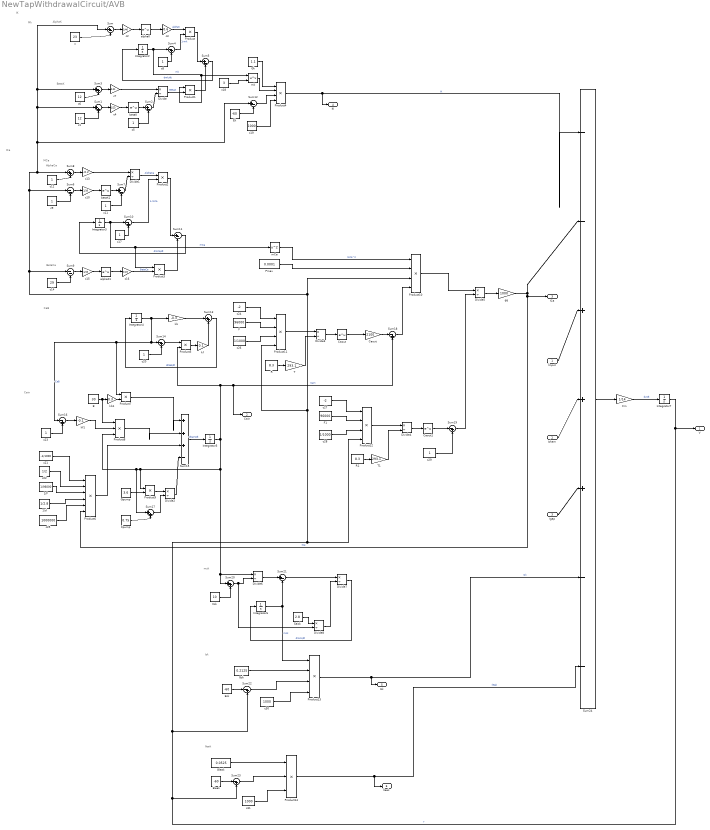
== system NewTapWithdrawalCircuit/AVB ==
  note: Isk
  note: msk
  note: ICa
  note: Cain
  note: CaB
  note: BetaCa
  note: AlphaCa
  note: MCa
  note: IK
  note: Mk
  note: BetaK
  note: AlphaK
  note: Ileak
  Iinput : Inport
  Ichem : Inport  Port=2
  Igap : Inport  Port=3
  1/F : Constant  Value=1/96000
  1/d : Constant  Value=1/2.8
  B : Constant  Value=30
  Caout : Math  SaturateOnIntegerOverflow=on
  "Caout " : Gain  Gain=2100
  Caout1 : Math  SaturateOnIntegerOverflow=on
  "Cm " : Gain  Gain=1/14
  Divide{,1..8} (9 alike) : Product  Inputs=*/
  "Ek " : Constant  Value=-60
  Eleak : Constant  Value=-60
  Esk : Constant  Value=-60
  F : Constant  Value=96000
  F1 : Constant  Value=96000
  "Gk " : Constant  Value=1.1
  Gleak : Constant  Value=0.0525
  Gpump : Constant  Value=3.6
  Gsk : Constant  Value=0.2125
  Integrator2 : Integrator
  Integrator3 : Integrator  InitialCondition=0.001
  Integrator4 : Integrator
  Integrator5 : Integrator
  Integrator6 : Integrator  InitialCondition=1
  Integrator7 : Integrator  InitialCondition=-60
  Kpump : Constant  Value=0.75
  Ksk : Constant  Value=10
  Pmax : Constant  Value=0.0001
  Product{,1..3,5,7,9} (7 alike) : Product
  Product{4,10..13} (5 alike) : Product  Inputs=4
  Product14 : Product  Inputs=3
  Product6 : Product  Inputs=6
  Product8 : Product  Inputs=3
  R : Constant  Value=8.3
  R1 : Constant  Value=8.3
  Saisk : Constant  Value=2.8
  Sum{,2,5,7,11..12,21} (7 alike) : Sum  Inputs=|+-
  Sum{1,3,8,13,17,20} (6 alike) : Sum  Inputs=|++
  Sum{4,10,14,16,18..19,22..23} (8 alike) : Sum  Inputs=|-+
  Sum15 : Sum  Inputs=|+++-
  Sum24 : Sum  Inputs=|--+++--
  Sum6 : Sum  Inputs=|--
  Sum9 : Sum  Inputs=|--
  T : Gain  Gain=293.1
  T1 : Gain  Gain=293.1
  alphaK : Math  SaturateOnIntegerOverflow=on
  alphaK1 : Math  SaturateOnIntegerOverflow=on
  betaK : Math  SaturateOnIntegerOverflow=on
  betaK1 : Math  SaturateOnIntegerOverflow=on
  c : Constant  Value=23
  c1 : Constant  Value=12
  c10 : Gain  Gain=1/10
  c{5,8..9,11..12,17,20,23,29} (9 alike) : Constant
  c13 : Gain  Gain=-0.2
  c14 : Constant  Value=29
  c15 : Gain  Gain=1/10
  c16 : Gain  Gain=0.23
  c18 : Constant  Value=3
  c19 : Constant  Value=1000
  c2 : Gain  Gain=1/46
  c21 : Constant  Value=-1/1000
  c22 : Constant  Value=1/2
  c24 : Constant  Value=-2
  c25 : Constant  Value=1000000
  c26 : Constant  Value=1/1000
  c27 : Constant  Value=-2
  c28 : Constant  Value=1/1000
  c3 : Gain  Gain=0.6
  c30 : Constant  Value=1000
  c31 : Constant  Value=1000
  c4 : Gain  Gain=1/23
  c6 : Constant  Value=12
  c7 : Gain  Gain=0.01
  "gg " : Gain  Gain=1000
  kb : Gain  Gain=-0.3
  kb1 : Gain  Gain=0.3
  kf : Gain  Gain=0.1
  kf1 : Gain  Gain=-0.1
  mCa : Math  Operator=square  SaturateOnIntegerOverflow=on
  mk : Math  Operator=pow  SaturateOnIntegerOverflow=on
  V : Outport
  "Cain " : Outport  Port=2
  ICa : Outport  Port=3
  IK : Outport  Port=4
  Isk : Outport  Port=5
  Ileak : Outport  Port=6
  wires:
  Divide/1 -> Product1/2  "BetaK"
  c10/1 -> betaK1/1
  Sum7/1 -> Divide1/2
  c/1 -> Sum/2
  R/1 -> T/1
  c3/1 -> Product/1  "alphaK"
  c9/1 -> Sum6/2
  c6/1 -> Sum3/2
  Product/1 -> Sum5/1
  Sum1/1 -> c4/1
  c13/1 -> Divide1/1
  Caout1/1 -> Sum19/1
  Eleak/1 -> Sum23/1
  T/1 -> Divide3/2
  Ksk/1 -> Sum20/2
  Product14/1 -> Ileak/1, Sum24/7  "Ileak"
  Sum24/1 -> "Cm "/1
  Esk/1 -> Sum22/1
  "Cm "/1 -> Integrator7/1  "dv/dt"
  Divide3/1 -> Caout/1
  c31/1 -> Product14/3
  Integrator6/1 -> Sum21/2, Product13/1  "msk"
  Sum21/1 -> Divide7/1
  Sum23/1 -> Product14/2
  Divide6/1 -> Sum21/1
  c12/1 -> Sum8/2
  Integrator3/1 -> Product3/1, mCa/1, Sum10/1  "mCa"
  Sum5/1 -> Integrator2/1  "dmk/dt"
  c15/1 -> alphaK1/1
  Sum9/1 -> c15/1
  c2/1 -> alphaK/1
  Sum22/1 -> Product13/3
  Product10/1 -> Divide5/1
  Integrator2/1 -> mk/1, Product1/1, Sum4/1  "mk"
  Divide8/1 -> Divide7/2
  R1/1 -> T1/1
  Caout/1 -> "Caout "/1
  Sum3/1 -> c7/1
  Sum6/1 -> c10/1
  Divide4/1 -> Caout1/1
  c30/1 -> Product13/4
  Gleak/1 -> Product14/1
  c28/1 -> Product12/3
  c11/1 -> Sum7/2
  betaK1/1 -> Sum7/1
  Divide7/1 -> Integrator6/1  "dmsk/dt"
  Ichem/1 -> Sum24/4
  c7/1 -> Divide/1
  Sum14/1 -> Product5/1
  Sum13/1 -> Integrator4/1  "dCaB/dt"
  Integrator5/1 -> Sum20/1, Divide6/1, Product9/1, Sum17/1, Product8/3, "Cain "/1, Sum18/2, Product5/2  "Cain"
  c21/1 -> Product6/1
  c22/1 -> Product6/2
  1/F/1 -> Product6/3
  1/d/1 -> Product6/4
  c25/1 -> Product6/5
  "gg "/1 -> Sum24/2, ICa/1, Product6/6  "ICa"
  B/1 -> Product8/1, kb1/1
  kb1/1 -> Product7/2
  Product7/1 -> Sum15/1
  Product5/1 -> kf/1
  kf/1 -> Sum13/2
  c23/1 -> Sum16/2
  Sum16/1 -> kf1/1
  kf1/1 -> Product8/2
  Product8/1 -> Sum15/2
  Product6/1 -> Sum15/3
  Gpump/1 -> Product9/2
  Product9/1 -> Divide2/1
  Kpump/1 -> Sum17/2
  Sum17/1 -> Divide2/2
  Divide2/1 -> Sum15/4
  Sum15/1 -> Integrator5/1  "dCain/dt"
  mCa/1 -> Product10/1  "mCa^2"
  Pmax/1 -> Product10/2
  c24/1 -> Product11/1
  F/1 -> Product11/2
  c26/1 -> Product11/3
  Integrator7/1 -> V/1, Sum22/2, Product11/4, Product10/3, Sum6/1, Sum1/1, Sum3/1, Sum/1, Sum12/1, Sum8/1, Sum9/1, Product12/4, Sum23/2  "v"
  c14/1 -> Sum9/2
  Saisk/1 -> Divide8/1
  Sum18/1 -> Product10/4
  Iinput/1 -> Sum24/3
  "Caout "/1 -> Sum18/1
  Sum/1 -> c2/1
  Sum8/1 -> c13/1
  c16/1 -> Product3/2  "BetaCa"
  Product11/1 -> Divide3/1
  T1/1 -> Divide4/2
  betaK/1 -> Sum2/1
  c29/1 -> Sum19/2
  Product1/1 -> Sum5/2
  c4/1 -> betaK/1
  alphaK/1 -> c3/1
  alphaK1/1 -> c16/1
  Divide1/1 -> Product2/1  "AlphaCa"
  Sum2/1 -> Divide/2
  Sum4/1 -> Product/2  "1-mk"
  c5/1 -> Sum2/2
  c8/1 -> Sum4/2
  Igap/1 -> Sum24/5
  Product13/1 -> Isk/1, Sum24/6  "Isk"
  Divide5/1 -> "gg "/1
  Sum20/1 -> Divide8/2, Divide6/2
  Gsk/1 -> Product13/2
  Product12/1 -> Divide4/1
  c27/1 -> Product12/1
  F1/1 -> Product12/2
  c1/1 -> Sum1/2
  Sum11/1 -> Integrator3/1  "dmCa/dt"
  c17/1 -> Sum10/2
  "Ek "/1 -> Sum12/2
  Sum10/1 -> Product2/2  "1-mCa"
  Sum12/1 -> Product4/3
  Product3/1 -> Sum11/2
  Product4/1 -> IK/1, Sum24/1  "IK"
  Integrator4/1 -> Product7/1, Sum16/1, Sum14/1, kb/1  "CaB"
  kb/1 -> Sum13/1
  c20/1 -> Sum14/2
  mk/1 -> Product4/2
  "Gk "/1 -> Product4/1
  c19/1 -> Product4/4
  Product2/1 -> Sum11/1
  c18/1 -> mk/2
  Sum19/1 -> Divide5/2
